simulink model "framesimulink"  (R2021b)
settings: Solver=ode3  StartTime=0.0  StopTime=5  FixedStep=Ts  RelTol=1e-3
model workspace (MAT data in the model file):
  Ts = 0.005
libraries: visionfilter x1, simulink x1
settings Model: Creator=GUBED49  LastModifiedBy=merciegu

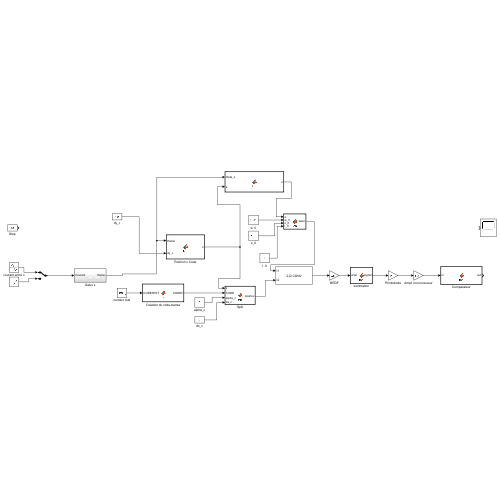
[thumbnail: Simulink's stored preview of the top-level diagram]
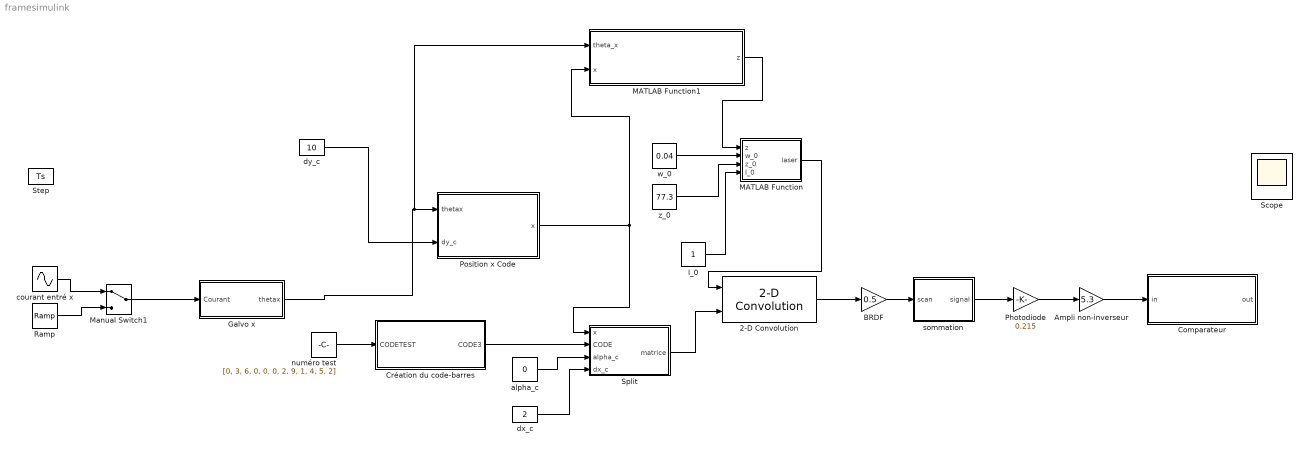
== system framesimulink ==
  2-D Convolution : visionfilter/2-D Convolution  outSize=Full  normalize=off  roundingMode=Floor  overflowMode=off  prodOutputMode=Binary point scaling  prodOutputWordLength=32  prodOutputFracLength=10  outputMode=Binary point scaling  outputWordLength=32  outputFracLength=12
      settings: SourceProductBaseCode=VP
  Ampli non-inverseur : Gain  Gain=5.3
  BRDF : Gain  Gain=0.5
  Comparateur : MATLAB Function  TreatAsAtomicUnit=on
  Création du code-barres : MATLAB Function  TreatAsAtomicUnit=on
  Galvo x : Subsystem
  I_0 : Constant
  MATLAB Function : MATLAB Function  TreatAsAtomicUnit=on
  MATLAB Function1 : MATLAB Function  TreatAsAtomicUnit=on
  Manual Switch1 : ManualSwitch
  Photodiode : Gain  Gain=0.215
  Position x Code : MATLAB Function  TreatAsAtomicUnit=on
  Ramp : simulink/Sources/Ramp  slope=20  start=0  InitialOutput=0
  Scope : Scope
  Split : MATLAB Function  TreatAsAtomicUnit=on
  Step : Constant  Value=Ts
  alpha_c : Constant  Value=0
  courant entré x : Sin  Amplitude=100  Frequency=5  SampleTime=0
  dx_c : Constant  Value=2
  dy_c : Constant  Value=10
  numéro test : Constant  Value=[0, 3, 6, 0, 0, 0, 2, 9, 1, 4, 5, 2]
  sommation : MATLAB Function  TreatAsAtomicUnit=on
  w_0 : Constant  Value=0.04
  z_0 : Constant  Value=77.3
  wires:
  MATLAB Function1/1(z) -> MATLAB Function/1(z)
  z_0/1 -> MATLAB Function/3(z_0)
  w_0/1 -> MATLAB Function/2(w_0)
  I_0/1 -> MATLAB Function/4(I_0)
  MATLAB Function/1(laser) -> 2-D Convolution/1
  numéro test/1 -> Création du code-barres/1(CODETEST)
  Manual Switch1/1 -> Galvo x/1(Courant)
  courant entré x/1 -> Manual Switch1/1
  Galvo x/1(" thetax") -> MATLAB Function1/1(theta_x), Position x Code/1(thetax)
  Ramp/1 -> Manual Switch1/2
  Création du code-barres/1(CODE3) -> Split/2(CODE)
  Split/1(matrice) -> 2-D Convolution/2
  dy_c/1 -> Position x Code/2(dy_c)
  Position x Code/1(x) -> Split/1(x), MATLAB Function1/2(x)
  alpha_c/1 -> Split/3(alpha_c)
  dx_c/1 -> Split/4(dx_c)
  2-D Convolution/1 -> BRDF/1
  BRDF/1 -> sommation/1(scan)
  sommation/1(signal) -> Photodiode/1
  Photodiode/1 -> Ampli non-inverseur/1
  Ampli non-inverseur/1 -> Comparateur/1(in)

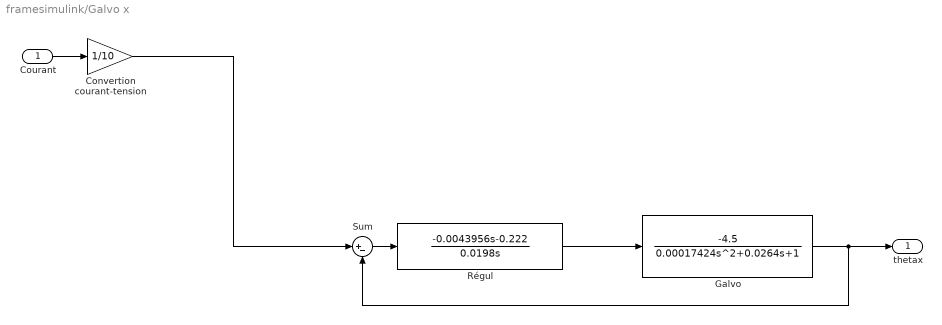
== system framesimulink/Galvo x ==
  Courant : Inport
  Convertion courant-tension : Gain  Gain=1/10
  "Galvo " : TransferFcn  Numerator=[-4.5]  Denominator="[0.00017424, 0.0264  1]"
  Régul : TransferFcn  Numerator=[-0.0043956, -0.222]  Denominator=[0.0198,0]
  Sum : Sum  Inputs=|+-
  " thetax" : Outport
  wires:
  Courant/1 -> Convertion courant-tension/1
  Convertion courant-tension/1 -> Sum/1
  Sum/1 -> Régul/1
  "Galvo "/1 -> " thetax"/1, Sum/2
  Régul/1 -> "Galvo "/1

== matlab function framesimulink/MATLAB Function1 ==
  data: theta_x input; x input; z output
function z = fcn(theta_x, x)

z=x/sind(theta_x);

== matlab function framesimulink/MATLAB Function ==
  data: z input; laser output; w_0 input; z_0 input; I_0 input
function laser = fcn(z, w_0, z_0, I_0)
pas=0.33;
laser4=zeros(4,4);
w = (w_0*sqrt(1+(z/z_0)^2));
for col= 1 : 4
    for row = 1 : 4
        col_1= (col*pas)-pas;
        row_1= (row*pas)-pas;
        rayon=sqrt(row_1^2+col_1^2);
laser4(row, col) = (I_0*(w_0/w)^(2)*exp((-2*((rayon)^2))/(w^2)));

    end
end
laser3=fliplr(laser4);
laser1=flipud(laser4);
laser2=fliplr(laser1);
laser=[laser2 laser1; laser3 laser4];

== matlab function framesimulink/Comparateur ==
  data: in input; out output
function out = fcn(in)
if in < 0
    in =
end

== matlab function framesimulink/Création du code-barres ==
  data: CODETEST input; CODE3 output
function CODE3 = fcn(CODETEST)
GAUCHE = [0 0 0 1 1 0 1; 0 0 1 1 0 0 1; 0 0 1 0 0 1 1; 0 1 1 1 1 0 1; 0 1 0 0 0 1 1; 0 1 1 0 0 0 1; 0 1 0 1 1 1 1; 0 1 1 1 0 1 1; 0 1 1 0 1 1 1; 0 0 0 1 0 1 1];
DROITE = [1 1 0 0 1 1 0; 1 1 0 1 1 0 0; 1 0 0 0 0 1 0; 1 0 1 1 1 0 0; 1 0 0 1 1 1 0; 1 0 1 0 0 0 0; 1 0 0 0 1 0 0; 1 0 0 1 0 0 0; 1 1 1 0 1 0 0; 1 1 1 0 0 1 0];

START=[ 1 0 1];
END=[1 0 1 0];
MIDDLE=[0 1 0 1 0];
CGAUCHE=[];
CDROITE=[];
QUIET=zeros(1,9);


for i = 1: 6
    val=CODETEST(i);
    val = val+1;
    CGAUCHE = [CGAUCHE;GAUCHE(val,:)];
end


for j = 7 : 12
    val=CODETEST(j);
    val = val+1;
    CDROITE = [CDROITE;DROITE(val,:)];
end 

CGAUCHE=transpose(CGAUCHE);
CGAUCHE=reshape(CGAUCHE,1,42);
CDROITE=transpose(CDROITE);
CDROITE=reshape(CDROITE,1,42);
CODE=[ QUIET START CGAUCHE MIDDLE CDROITE END QUIET];
CODEBAS= [ QUIET START zeros([1 42]) MIDDLE zeros([1 42]) END QUIET];


for i=1:77
    CODE2=[CODE;CODE(1,:)];
end
for i=1:5
    CODE3=[CODE2;CODEBAS(1,:)];
end

== matlab function framesimulink/sommation ==
  data: scan input; signal output
function signal = fcn(scan)
signal=sum(sum(scan(:)));

== matlab function framesimulink/Position x Code ==
  data: thetax input; x output; dy_c input
function x  = fcn(thetax,dy_c)
x = (tand(thetax)*dy_c);

== matlab function framesimulink/Split ==
  data: x input; CODE input; matrice output; alpha_c input; dx_c input
function matrice  = fcn(x, CODE, alpha_c, dx_c)

c =(x/cosd(alpha_c)) ;
c_1 = round(c/0.033);
if c_1 > 53 
c_1 = 53;
end
if c_1 < - 53
    c_1 = -53;
end
matrice = CODE(:,54+c_1);
